simulink model "Modele_causal"  (R2023a)
settings: Solver=VariableStepAuto  StartTime=0.0  StopTime=10  RelTol=1e-3
values from neighbouring files (symbols this model uses):
  f = 0    [parametres.m]
  Imax = 4.3    [parametres.m]
  K_codeur = 23    [parametres.m]
  K_meca = 0.01    [parametres.m]
  Kc = 52.5e-3    (= 0.0525)    [parametres.m]
  KD_p = 15000    [parametres.m]
  Ke = 1/(182*2*pi/60)    (= 0.0524686625578)    [parametres.m]
  KI_i = 200    [parametres.m]
  KI_p = 4800    [parametres.m]
  KP_i = 800    [parametres.m]
  KP_p = 5600    [parametres.m]
  Lm = 0.62e-3    (= 0.00062)    [parametres.m]
  Rm = 2.07    [parametres.m]
  t_acc = theta_p / theta_pp    (= 0.277777777778)    [parametres.m]
  theta_p = 2.5    [parametres.m]
  Umax = 24    [parametres.m]
undefined symbols (not defined in the file or in its folder): Jeq
libraries: simulink x4
settings Model: Creator=xpess  LastModifiedBy=xpess

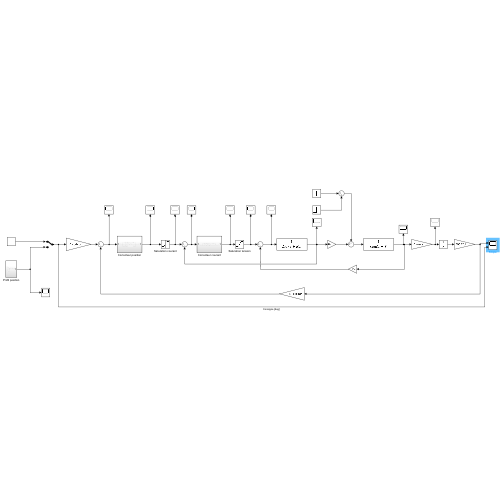
[thumbnail: Simulink's stored preview of the top-level diagram]
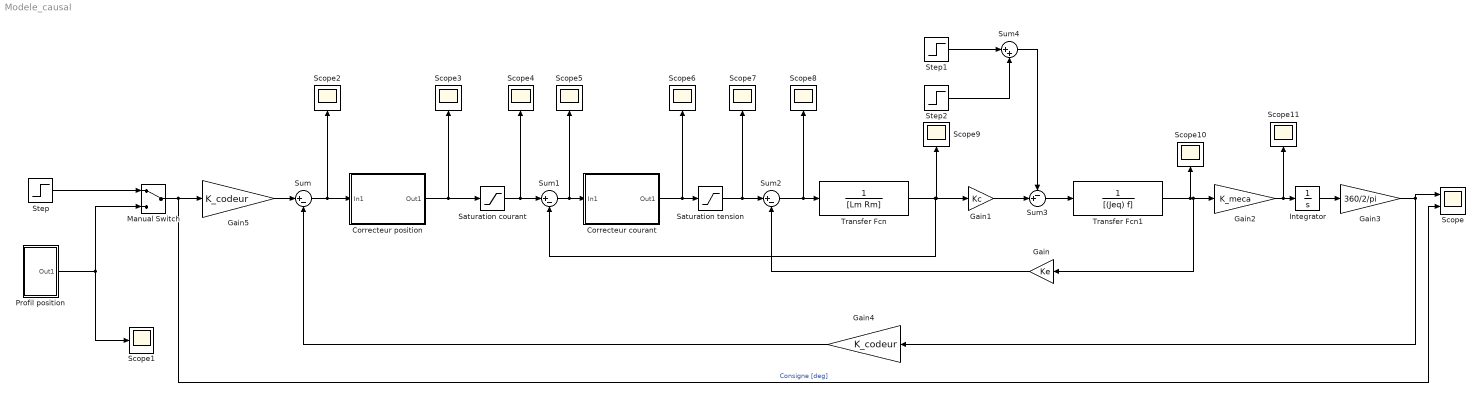
== system Modele_causal ==
  Correcteur courant : Subsystem
  Correcteur position : Subsystem
  Gain : Gain  Gain=Ke
  Gain1 : Gain  Gain=Kc
  Gain2 : Gain  Gain=K_meca
  Gain3 : Gain  Gain=360/2/pi
  Gain4 : Gain  Gain=K_codeur
  Gain5 : Gain  Gain=K_codeur
  Integrator : Integrator
  Manual Switch : ManualSwitch
  Profil position : Subsystem
  Saturation courant : Saturate  UpperLimit=Imax  LowerLimit=-Imax
  Saturation tension : Saturate  UpperLimit=Umax  LowerLimit=-Umax
  Scope : Scope  NumInputPorts=2
  Scope{1..11} (11 alike) : Scope
  Step : Step  Time=0  After=10  SampleTime=0
  Step1 : Step  After=0  SampleTime=0
  Step2 : Step  After=0  SampleTime=0
  Sum : Sum  Inputs=|+-
  Sum1 : Sum  Inputs=|+-
  Sum2 : Sum  Inputs=|+-
  Sum3 : Sum  Inputs=-+|
  Sum4 : Sum  Inputs=|++
  Transfer Fcn : TransferFcn  Denominator=[Lm Rm]
  Transfer Fcn1 : TransferFcn  Denominator=[(Jeq) f]
  wires:
  Sum/1 -> Correcteur position/1(In1), Scope2/1
  Correcteur position/1(Out1) -> Saturation courant/1, Scope3/1
  Correcteur courant/1(Out1) -> Scope6/1, Saturation tension/1
  Sum1/1 -> Scope5/1, Correcteur courant/1(In1)
  Saturation courant/1 -> Scope4/1, Sum1/1
  Saturation tension/1 -> Sum2/1, Scope7/1
  Sum2/1 -> Scope8/1, Transfer Fcn/1
  Transfer Fcn/1 -> Scope9/1, Gain1/1, Sum1/2
  Transfer Fcn1/1 -> Gain/1, Gain2/1, Scope10/1
  Gain/1 -> Sum2/2
  Integrator/1 -> Gain3/1
  Sum3/1 -> Transfer Fcn1/1
  Gain1/1 -> Sum3/2
  Gain3/1 -> Scope/1, Gain4/1
  Step2/1 -> Sum4/2
  Step1/1 -> Sum4/1
  Sum4/1 -> Sum3/1
  Gain4/1 -> Sum/2
  Gain5/1 -> Sum/1
  Step/1 -> Manual Switch/1
  Profil position/1(Out1) -> Manual Switch/2, Scope1/1
  Manual Switch/1 -> Scope/2, Gain5/1  "Consigne [deg]"
  Gain2/1 -> Scope11/1, Integrator/1

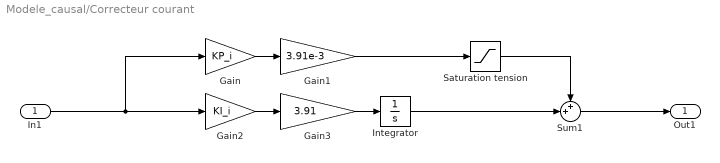
== system Modele_causal/Correcteur courant ==
  In1 : Inport
  Gain : Gain  Gain=KP_i
  Gain1 : Gain  Gain=3.91e-3
  Gain2 : Gain  Gain=KI_i
  Gain3 : Gain  Gain=3.91
  Integrator : Integrator
  Saturation tension : Saturate  UpperLimit=Umax  LowerLimit=-Umax
  Sum1 : Sum  Inputs=++|
  Out1 : Outport
  wires:
  Sum1/1 -> Out1/1
  Gain3/1 -> Integrator/1
  Integrator/1 -> Sum1/2
  Gain2/1 -> Gain3/1
  In1/1 -> Gain2/1, Gain/1
  Gain/1 -> Gain1/1
  Gain1/1 -> Saturation tension/1
  Saturation tension/1 -> Sum1/1

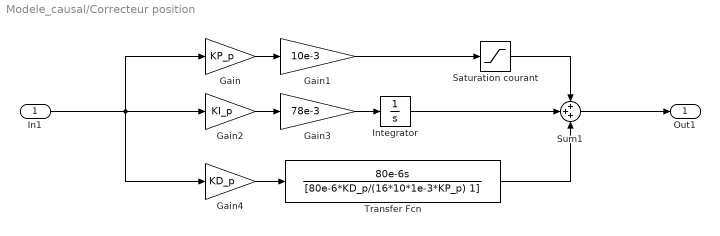
== system Modele_causal/Correcteur position ==
  In1 : Inport
  Gain : Gain  Gain=KP_p
  Gain1 : Gain  Gain=10e-3
  Gain2 : Gain  Gain=KI_p
  Gain3 : Gain  Gain=78e-3
  Gain4 : Gain  Gain=KD_p
  Integrator : Integrator
  Saturation courant : Saturate  UpperLimit=Imax  LowerLimit=-Imax
  Sum1 : Sum  Inputs=+++
  Transfer Fcn : TransferFcn  Numerator=[80e-6 0]  Denominator=[80e-6*KD_p/(16*10*1e-3*KP_p) 1]
  Out1 : Outport
  wires:
  Transfer Fcn/1 -> Sum1/3
  Gain1/1 -> Saturation courant/1
  Gain/1 -> Gain1/1
  In1/1 -> Gain/1, Gain4/1, Gain2/1
  Gain2/1 -> Gain3/1
  Integrator/1 -> Sum1/2
  Gain4/1 -> Transfer Fcn/1
  Gain3/1 -> Integrator/1
  Sum1/1 -> Out1/1
  Saturation courant/1 -> Sum1/1

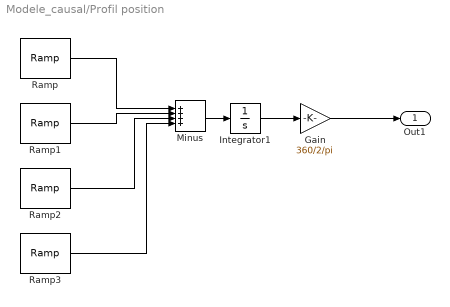
== system Modele_causal/Profil position ==
  Gain : Gain  Gain=360/2/pi
  Integrator1 : Integrator
  Minus : Sum  Inputs=++++
  Ramp : simulink/Sources/Ramp  slope=theta_p/t_acc  start=t0  InitialOutput=0
  Ramp1 : simulink/Sources/Ramp  slope=-theta_p/t_acc  start=t1  InitialOutput=0
  Ramp2 : simulink/Sources/Ramp  slope=-theta_p/t_acc  start=t2  InitialOutput=0
  Ramp3 : simulink/Sources/Ramp  slope=theta_p/t_acc  start=t3  InitialOutput=0
  Out1 : Outport
  wires:
  Ramp/1 -> Minus/1
  Integrator1/1 -> Gain/1
  Ramp3/1 -> Minus/4
  Ramp1/1 -> Minus/2
  Ramp2/1 -> Minus/3
  Minus/1 -> Integrator1/1
  Gain/1 -> Out1/1
